simulink model "PlannedIsland"  (R2025a)
settings: Solver=FixedStepAuto  StartTime=0.0  StopTime=10.0  RelTol=1e-3
model mask{KpPPlannedIsland=KpPPlannedIsland, KiPPlannedIsland=KiPPlannedIsland, ZeroActivePowerThreshold=ZeroActivePowerThreshold, KpQPlannedIsland=KpQPlannedIsland, KiQPlannedIsland=KiQPlannedIsland, ZeroReactivePowerThreshold=ZeroReactivePowerThreshold}
  mask prompts: KpPPlannedIsland "Proportional Gain"; KiPPlannedIsland "Integral Gain"; ZeroActivePowerThreshold "Threshold"; KpQPlannedIsland "Proportional Gain"; KiQPlannedIsland "Integral Gain"; ZeroReactivePowerThreshold "Threshold"
model workspace (MAT data in the model file):
  KiPPlannedIsland = 1
  KiQPlannedIsland = 0
  KpPPlannedIsland = 1
  KpQPlannedIsland = 1
  Ts = 0.001
  ZeroActivePowerThreshold = 0.001
  ZeroReactivePowerThreshold = 0.001
libraries: slpidlib x2, eeGeneralControl x1
settings Model: ParameterArgumentNames=KiPPlannedIsland,KiQPlannedIsland,KpPPlannedIsland,KpQPlannedIsland,ZeroActivePowerThreshold,ZeroReactivePowerThreshold  Creator=skota  LastModifiedBy=skota
settings DataIOCC: SaveFormat=StructureWithTime  SaveOutput=off  SignalLogging=off  DSMLogging=off  SaveTime=off  ReturnWorkspaceOutputs=off
settings RTWCC: Toolchain=MinGW64 | CMake/gmake (64-bit Windows)  BuildConfiguration=Release  GPUComputeCapability=3.5

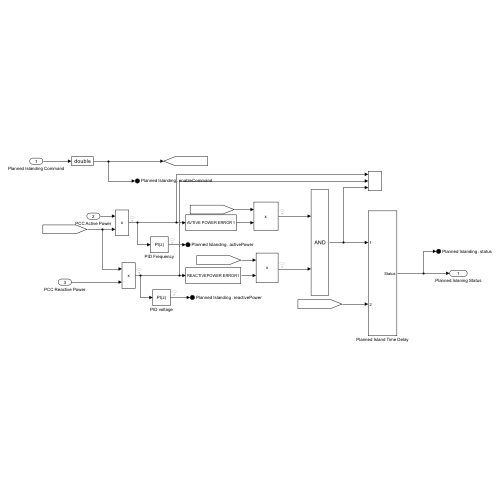
[thumbnail: Simulink's stored preview of the top-level diagram]
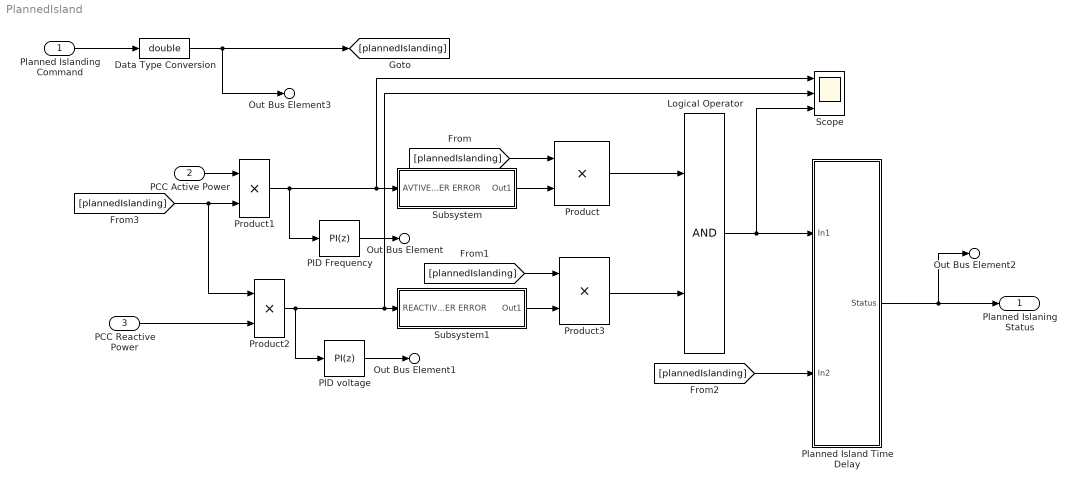
== system PlannedIsland ==
  Planned Islanding Command : Inport  OutDataTypeStr=boolean
  PCC Active Power : Inport  Port=2
  PCC Reactive Power : Inport  Port=3
  Data Type Conversion : DataTypeConversion  OutDataTypeStr=double  SaturateOnIntegerOverflow=off  RndMeth=Floor
  Logical Operator : Logic  AllPortsSameDT=off  OutDataTypeStr=boolean
  PID Frequency : slpidlib/PID Controller  Controller=PI  Form=Parallel  TimeDomain=Discrete-time  UseExternalTs=off  SampleTime=Ts  IntegratorMethod=Forward Euler  FilterMethod=Forward Euler  ControllerParametersSource=internal  P=KpPPlannedIsland  I=KiPPlannedIsland  UseKiTs=off  D=0  UseExternalDerivativeSource=off  N=100  UseFilter=on  TunerSelectOption=Frequency Response Based  InitialConditionSource=internal  InitialConditionForIntegrator=0  InitialConditionForFilter=0  DifferentiatorICPrevScaledInput=0  ExternalReset=none  TrackingMode=off  Kt=1  LimitOutput=off  SatLimitsSource=internal  UpperSaturationLimit=0.05  LowerSaturationLimit=-0.05  LinearizeAsGain=on  AntiWindupMode=clamping  Kb=1  LimitIntegrator=off  UpperIntegratorSaturationLimit=inf  LowerIntegratorSaturationLimit=-inf  POutMin=[]  POutMax=[]  IOutMin=[]  IOutMax=[]  DOutMin=[]  DOutMax=[]  NOutMin=[]  NOutMax=[]  SumOutMin=[]  SumOutMax=[]  SaturationOutMin=[]  SaturationOutMax=[]  PParamMin=[]  PParamMax=[]  IParamMin=[]  IParamMax=[]  DParamMin=[]  DParamMax=[]  NParamMin=[]  NParamMax=[]  KbParamMin=[]  KbParamMax=[]  KtParamMin=[]  KtParamMax=[]  KbOutMin=[]  KbOutMax=[]  KtOutMin=[]  KtOutMax=[]  IntegratorOutMin=[]  IntegratorOutMax=[]  FilterOutMin=[]  FilterOutMax=[]  SumI1OutMin=[]  SumI1OutMax=[]  SumI2OutMin=[]  SumI2OutMax=[]  SumI3OutMin=[]  SumI3OutMax=[]  SumI4OutMin=[]  SumI4OutMax=[]  SumDOutMin=[]  SumDOutMax=[]  DifferentiatorOutMin=[]  DifferentiatorOutMax=[]  FilterDiffOutCoefMin=[]  FilterDiffOutCoefMax=[]  ReciprocalOutMin=[]  ReciprocalOutMax=[]  SumDenOutMin=[]  SumDenOutMax=[]  SumNumOutMin=[]  SumNumOutMax=[]  DivideOutMin=[]  DivideOutMax=[]  UdiffTsProdOutMin=[]  UdiffTsProdOutMax=[]  NTsProdOutMin=[]  NTsProdOutMax=[]  UintegralTsProdOutMin=[]  UintegralTsProdOutMax=[]  UngainTsProdOutMin=[]  UngainTsProdOutMax=[]  ClampingZeroOutDataTypeStr=Inherit: Inherit via back propagation  ClampingZeroOutMin=[]  ClampingZeroOutMax=[]  FilterDenConstantOutDataTypeStr=Inherit: Inherit via back propagation  FilterDenConstantOutMin=[]  FilterDenConstantOutMax=[]  PCopyOutDataTypeStr=Inherit: Inherit via back propagation  PCopyOutMin=[]  PCopyOutMax=[]  NCopyOutDataTypeStr=Inherit: Inherit via back propagation  NCopyOutMin=[]  NCopyOutMax=[]  IntegratorContinuousStateAttributes=''  IntegratorStateMustResolveToSignalObject=off  IntegratorRTWStateStorageClass=Auto  FilterContinuousStateAttributes=''  FilterStateMustResolveToSignalObject=off  FilterRTWStateStorageClass=Auto  ParallelPVariant=InternalParameters  IdealPVariant=Disabled  IVariant=InternalParameters  DVariant=Disabled  IntegratorVariant=Discrete  SatVariant=Disabled  AWVariant=Passthrough  PCopyVariant=Disabled  TRVariant=Disabled  FdbkBlocksVariant=Forward  IdealPFdbkVariant=Disabled  SatFdbkVariant=Disabled  DerivativeFilterVariant=Disabled  NVariant=Disabled  NCopyVariant=Disabled_SignalSpec  FilterICVariant=Disabled  IntegratorICVariant=InternalICs  ExternalResetVariant=Disabled  TRSumVariant=Passthrough  SumFdbkVariant=Disabled  SumVariant=Sum_PI  TsampFilterVariant=InternalTs  TsampNgainVariant=Passthrough  TsampIntegralVariant=Disabled_SignalSpec  ExternalSaturationOutDataTypeStr=Inherit: Same as second input  DerivativeSourceVariant=Disabled  PreIntVariant=InternalPreInt
  PID voltage : slpidlib/PID Controller  Controller=PI  Form=Parallel  TimeDomain=Discrete-time  UseExternalTs=off  SampleTime=Ts  IntegratorMethod=Forward Euler  FilterMethod=Forward Euler  ControllerParametersSource=internal  P=KpQPlannedIsland  I=KiQPlannedIsland  UseKiTs=off  D=0  UseExternalDerivativeSource=off  N=100  UseFilter=on  TunerSelectOption=Frequency Response Based  InitialConditionSource=internal  InitialConditionForIntegrator=0  InitialConditionForFilter=0  DifferentiatorICPrevScaledInput=0  ExternalReset=none  TrackingMode=off  Kt=1  LimitOutput=off  SatLimitsSource=internal  UpperSaturationLimit=0.05  LowerSaturationLimit=-0.05  LinearizeAsGain=on  AntiWindupMode=clamping  Kb=1  LimitIntegrator=off  UpperIntegratorSaturationLimit=inf  LowerIntegratorSaturationLimit=-inf  POutMin=[]  POutMax=[]  IOutMin=[]  IOutMax=[]  DOutMin=[]  DOutMax=[]  NOutMin=[]  NOutMax=[]  SumOutMin=[]  SumOutMax=[]  SaturationOutMin=[]  SaturationOutMax=[]  PParamMin=[]  PParamMax=[]  IParamMin=[]  IParamMax=[]  DParamMin=[]  DParamMax=[]  NParamMin=[]  NParamMax=[]  KbParamMin=[]  KbParamMax=[]  KtParamMin=[]  KtParamMax=[]  KbOutMin=[]  KbOutMax=[]  KtOutMin=[]  KtOutMax=[]  IntegratorOutMin=[]  IntegratorOutMax=[]  FilterOutMin=[]  FilterOutMax=[]  SumI1OutMin=[]  SumI1OutMax=[]  SumI2OutMin=[]  SumI2OutMax=[]  SumI3OutMin=[]  SumI3OutMax=[]  SumI4OutMin=[]  SumI4OutMax=[]  SumDOutMin=[]  SumDOutMax=[]  DifferentiatorOutMin=[]  DifferentiatorOutMax=[]  FilterDiffOutCoefMin=[]  FilterDiffOutCoefMax=[]  ReciprocalOutMin=[]  ReciprocalOutMax=[]  SumDenOutMin=[]  SumDenOutMax=[]  SumNumOutMin=[]  SumNumOutMax=[]  DivideOutMin=[]  DivideOutMax=[]  UdiffTsProdOutMin=[]  UdiffTsProdOutMax=[]  NTsProdOutMin=[]  NTsProdOutMax=[]  UintegralTsProdOutMin=[]  UintegralTsProdOutMax=[]  UngainTsProdOutMin=[]  UngainTsProdOutMax=[]  ClampingZeroOutDataTypeStr=Inherit: Inherit via back propagation  ClampingZeroOutMin=[]  ClampingZeroOutMax=[]  FilterDenConstantOutDataTypeStr=Inherit: Inherit via back propagation  FilterDenConstantOutMin=[]  FilterDenConstantOutMax=[]  PCopyOutDataTypeStr=Inherit: Inherit via back propagation  PCopyOutMin=[]  PCopyOutMax=[]  NCopyOutDataTypeStr=Inherit: Inherit via back propagation  NCopyOutMin=[]  NCopyOutMax=[]  IntegratorContinuousStateAttributes=''  IntegratorStateMustResolveToSignalObject=off  IntegratorRTWStateStorageClass=Auto  FilterContinuousStateAttributes=''  FilterStateMustResolveToSignalObject=off  FilterRTWStateStorageClass=Auto  ParallelPVariant=InternalParameters  IdealPVariant=Disabled  IVariant=InternalParameters  DVariant=Disabled  IntegratorVariant=Discrete  SatVariant=Disabled  AWVariant=Passthrough  PCopyVariant=Disabled  TRVariant=Disabled  FdbkBlocksVariant=Forward  IdealPFdbkVariant=Disabled  SatFdbkVariant=Disabled  DerivativeFilterVariant=Disabled  NVariant=Disabled  NCopyVariant=Disabled_SignalSpec  FilterICVariant=Disabled  IntegratorICVariant=InternalICs  ExternalResetVariant=Disabled  TRSumVariant=Passthrough  SumFdbkVariant=Disabled  SumVariant=Sum_PI  TsampFilterVariant=InternalTs  TsampNgainVariant=Passthrough  TsampIntegralVariant=Disabled_SignalSpec  ExternalSaturationOutDataTypeStr=Inherit: Same as second input  DerivativeSourceVariant=Disabled  PreIntVariant=InternalPreInt
  Planned Island Time Delay : Subsystem
  Product{,1..3} (4 alike) : Product
  Scope : Scope  NumInputPorts=3
  Subsystem : Subsystem
  Subsystem1 : Subsystem
  Planned Islaning Status : Outport
  Out Bus Element : Outport  Port=2  PortName=Planned Islanding  Element=activePower
  Out Bus Element1 : Outport  Port=2  PortName=Planned Islanding  Element=reactivePower
  Out Bus Element2 : Outport  Port=2  PortName=Planned Islanding  Element=status
  Out Bus Element3 : Outport  Port=2  PortName=Planned Islanding  Element=enableCommand
  wires:
  [plannedIslanding] -> Product3/1
  [plannedIslanding] -> Product/1
  Subsystem/1(Out1) -> Product/2
  Planned Islanding Command/1 -> Data Type Conversion/1
  PCC Reactive Power/1 -> Product2/2
  Product/1 -> Logical Operator/1
  Product3/1 -> Logical Operator/2
  Planned Island Time Delay/1(Status) -> Out Bus Element2/1, Planned Islaning Status/1
  PID Frequency/1 -> Out Bus Element/1
  Logical Operator/1 -> Scope/3, Planned Island Time Delay/1(In1)
  PID voltage/1 -> Out Bus Element1/1
  [plannedIslanding] -> Planned Island Time Delay/2(In2)
  Subsystem1/1(Out1) -> Product3/2
  PCC Active Power/1 -> Product1/1
  [plannedIslanding] -> Product2/1, Product1/2
  Product1/1 -> PID Frequency/1, Scope/1, Subsystem/1(AVTIVE POWER ERROR)
  Data Type Conversion/1 -> Out Bus Element3/1, [plannedIslanding]
  Product2/1 -> PID voltage/1, Scope/2, Subsystem1/1(REACTIVEPOWER ERROR)

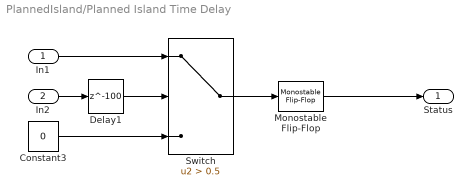
== system PlannedIsland/Planned Island Time Delay ==
  In1 : Inport
  In2 : Inport  Port=2
  Constant3 : Constant  Value=0
  Delay1 : Delay  DelayLength=100  SampleTime=Ts
  Monostable Flip-Flop : eeGeneralControl/Monostable Flip-Flop  VariantControl=Variant1  LabelModeActiveChoice=Discrete  ChangeType=Rising edge  x0=0  Td=100  Ts=Ts
      settings: LibrarySourceBlock=ee_sl_lib/General Control/Monostable Flip-Flop
  Switch : Switch  Criteria=u2 > Threshold  Threshold=0.5  SaturateOnIntegerOverflow=off  InputSameDT=off
  Status : Outport
  wires:
  In2/1 -> Delay1/1
  In1/1 -> Switch/1
  Monostable Flip-Flop/1 -> Status/1
  Delay1/1 -> Switch/2
  Constant3/1 -> Switch/3
  Switch/1 -> Monostable Flip-Flop/1

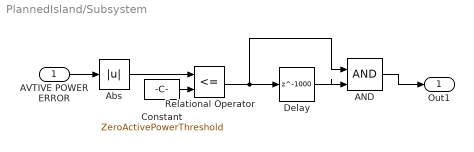
== system PlannedIsland/Subsystem ==
  AVTIVE POWER ERROR : Inport
  AND : Logic  IconShape=distinctive  AllPortsSameDT=off  OutDataTypeStr=boolean
  Abs : Abs  SaturateOnIntegerOverflow=off
  Constant : Constant  Value=ZeroActivePowerThreshold  SampleTime=-1
  Delay : Delay  DelayLength=1000  SampleTime=Ts
  Relational Operator : RelationalOperator  Operator=<=  OutDataTypeStr=boolean  RndMeth=Simplest  InputSameDT=off
  Out1 : Outport
  wires:
  Delay/1 -> AND/2
  Constant/1 -> Relational Operator/2
  Relational Operator/1 -> AND/1, Delay/1
  AND/1 -> Out1/1
  AVTIVE POWER ERROR/1 -> Abs/1
  Abs/1 -> Relational Operator/1

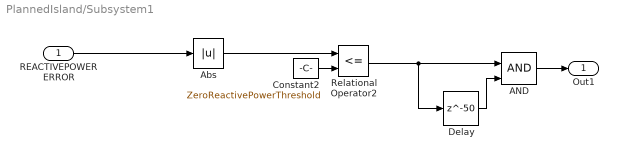
== system PlannedIsland/Subsystem1 ==
  REACTIVEPOWER ERROR : Inport
  AND : Logic  IconShape=distinctive  AllPortsSameDT=off  OutDataTypeStr=boolean
  Abs : Abs  SaturateOnIntegerOverflow=off
  Constant2 : Constant  Value=ZeroReactivePowerThreshold
  Delay : Delay  DelayLength=50  SampleTime=Ts
  Relational Operator2 : RelationalOperator  Operator=<=  OutDataTypeStr=boolean  RndMeth=Simplest  InputSameDT=off
  Out1 : Outport
  wires:
  Delay/1 -> AND/2
  REACTIVEPOWER ERROR/1 -> Abs/1
  Relational Operator2/1 -> Delay/1, AND/1
  Constant2/1 -> Relational Operator2/2
  AND/1 -> Out1/1
  Abs/1 -> Relational Operator2/1
